simulink model "LinearMPC_pH"  (R2018a)
settings: Solver=ode45  StartTime=0.0  StopTime=10000  RelTol=1e-3  EnableMultiTasking=on
undefined symbols (not defined in the file or in its folder): sigbuilder_block
libraries: mpclib x1, simulink x1
settings Model: Creator=Debbie Ojigho  LastModifiedBy=Owolabi Israel
settings DataIOCC: LimitDataPoints=on  SaveFormat=Array
settings OptimizationCC: LifeSpan=inf
settings DebuggingCC: SFUnexpectedBacktrackingDiag=warning  SFNoUnconditionalDefaultTransitionDiag=warning  SFExecutionAtInitializationDiag=none
settings HardwareCC: ProdBitPerPointer=32  ProdBitPerSizeT=32  ProdBitPerPtrDiffT=32  ProdLargestAtomicFloat=None  ProdIntDivRoundTo=Undefined  ProdEndianess=Unspecified  ProdWordSize=32  ProdHWDeviceType=32-bit Generic
settings ModelReferenceCC: PropagateSignalLabelsOutOfModel=off
settings CodeAppCC: StateflowObjectComments=on
settings GRTTargetCC: TargetLangStandard=C89/C90 (ANSI)  GeneratePreprocessorConditionals=Disable all
settings ConfigComp: CovMetricSettings=dw  CovHtmlReporting=on  CovSaveCumulativeToWorkspaceVar=on  CovSaveSingleToWorkspaceVar=on  CovExternalEMLEnable=off

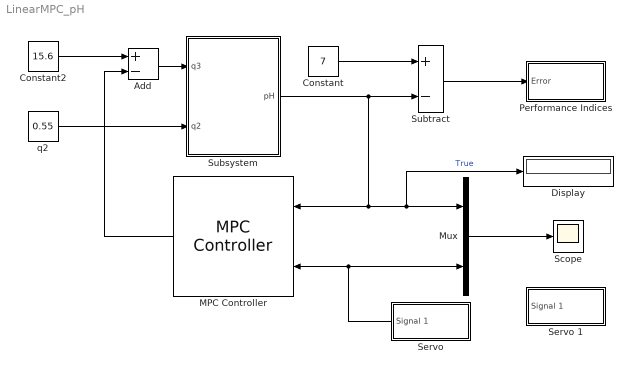
== system LinearMPC_pH ==
  Add : Sum  Inputs=+-
  Constant : Constant  Value=7
  Constant2 : Constant  Value=15.6
  Display : Display
  MPC Controller : mpclib/MPC Controller  SCDEnableBlockLinearizationSpecification=on  mpcobj=mpcobj_pH  x0=[]  is_multiple=0  enable_value=0  return_u0=off  updateMPCinCallerWorkspace=on  md_inport=off  mv_inport=off  uref_inport=off  cost_outport=off  return_sequence=off  return_qpstatus=off  return_xseq=off  return_state=off  return_ovseq=off  state_inport=off  umin_inport=off  umax_inport=off  ymin_inport=off  ymax_inport=off  cc_inport=off  ywt_inport=off  uwt_inport=off  duwt_inport=off  rhoeps_inport=off  pm_inport=off  MaximumP=10  HorizonChoice=FixedHorizon  n_ts=1  n_p=3  n_mv=1  n_md=0  n_ud=0  n_mo=1  n_uo=0  BlockDataType=double  SampleTimeInherited=off  switch_inport=off
      settings: SourceProductName=MATLAB Runtime - Model Predictive Control Toolbox Addin  SourceProductBaseCode=Missing
  Mux : Mux  Inputs=2
  Performance Indices : Subsystem
  Scope : Scope
  "Servo " : Subsystem  Tag=STV Subsys  LoadFcn=sigbuilder_block('load');  StartFcn=sigbuilder_block('start');  StopFcn=sigbuilder_block('stop');  ClipboardFcn=sigbuilder_block('clipboard');  mask(Sigbuilder block){tuvar=[0:10]}
      mask help: Sigbuilder GUI
      mask init:
      | if ~strcmp(get_param(bdroot(gcbh),'SimulationStatus'),'stopped') tuvar = sigbuilder_block('maskInit'); end
      settings: CopyFcn=sigbuilder_block('copy');  DeleteFcn=sigbuilder_block('delete');  ModelCloseFcn=sigbuilder_block('modelClose');  PreSaveFcn=sigbuilder_block('preSave');  PauseFcn=sigbuilder_block('pause')  ContinueFcn=sigbuilder_block('continue')  NameChangeFcn=sigbuilder_block('namechange');  OpenFcn=sigbuilder_block('open',[203.25 112.5 550.5 399.75 ]);  CloseFcn=sigbuilder_block('close');
      mask Display: plot(0, 0, 100, 100,[2, 2, 32, 32, 2], [68, 8, 8, 68, 68],[32, 2], [38, 38], [32, 19, 2],[53, 60, 44], [32, 17, 17, 2],[16, 16, 31, 31]);txt = getActiveGroup(gcbh);text(2, 100, txt,'verticalAlignment', 'top');
  Servo 1 : Subsystem  Tag=STV Subsys  LoadFcn=sigbuilder_block('load');  StartFcn=sigbuilder_block('start');  StopFcn=sigbuilder_block('stop');  ClipboardFcn=sigbuilder_block('clipboard');  mask(Sigbuilder block){tuvar=[0:10]}
      mask help: Sigbuilder GUI
      mask init:
      | if ~strcmp(get_param(bdroot(gcbh),'SimulationStatus'),'stopped') tuvar = sigbuilder_block('maskInit'); end
      settings: CopyFcn=sigbuilder_block('copy');  DeleteFcn=sigbuilder_block('delete');  ModelCloseFcn=sigbuilder_block('modelClose');  PreSaveFcn=sigbuilder_block('preSave');  PauseFcn=sigbuilder_block('pause')  ContinueFcn=sigbuilder_block('continue')  NameChangeFcn=sigbuilder_block('namechange');  OpenFcn=sigbuilder_block('open',[203.25 112.5 550.5 399.75 ]);  CloseFcn=sigbuilder_block('close');
      mask Display: plot(0, 0, 100, 100,[2, 2, 32, 32, 2], [68, 8, 8, 68, 68],[32, 2], [38, 38], [32, 19, 2],[53, 60, 44], [32, 17, 17, 2],[16, 16, 31, 31]);txt = getActiveGroup(gcbh);text(2, 100, txt,'verticalAlignment', 'top');
  Subsystem : Subsystem
  Subtract : Sum  Inputs=+-
  q2 : Constant  Value=0.55
  wires:
  Subtract/1 -> Performance Indices/1("Error ")
  Mux/1 -> Scope/1
  Subsystem/1(pH) -> Subtract/2, MPC Controller/1, Display/1, Mux/1  "True"
  Constant/1 -> Subtract/1
  "Servo "/1(Signal 1) -> MPC Controller/2, Mux/2
  q2/1 -> Subsystem/2(q2)
  Add/1 -> Subsystem/1(q3)
  Constant2/1 -> Add/1
  MPC Controller/1 -> Add/2

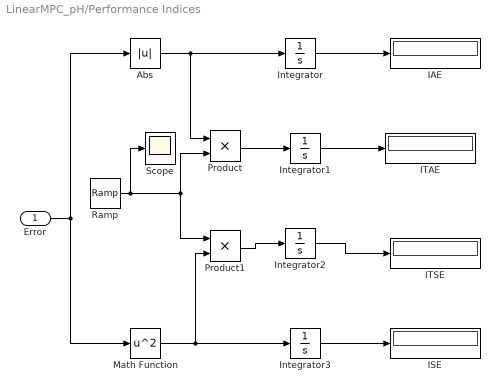
== system LinearMPC_pH/Performance Indices ==
  "Error " : Inport
  Abs : Abs
  IAE : Display
  ISE : Display
  ITAE : Display
  ITSE : Display
  Integrator{,1..3} (4 alike) : Integrator
  Math Function : Math  Operator=square  SaturateOnIntegerOverflow=on
  Product : Product  RndMeth=Zero
  Product1 : Product  RndMeth=Zero
  Ramp : simulink/Sources/Ramp  slope=1  start=0  InitialOutput=0
  Scope : Scope
  wires:
  "Error "/1 -> Math Function/1, Abs/1
  Abs/1 -> Integrator/1, Product/1
  Integrator/1 -> IAE/1
  Ramp/1 -> Product/2, Product1/1, Scope/1
  Math Function/1 -> Integrator3/1, Product1/2
  Product1/1 -> Integrator2/1
  Product/1 -> Integrator1/1
  Integrator3/1 -> ISE/1
  Integrator2/1 -> ITSE/1
  Integrator1/1 -> ITAE/1

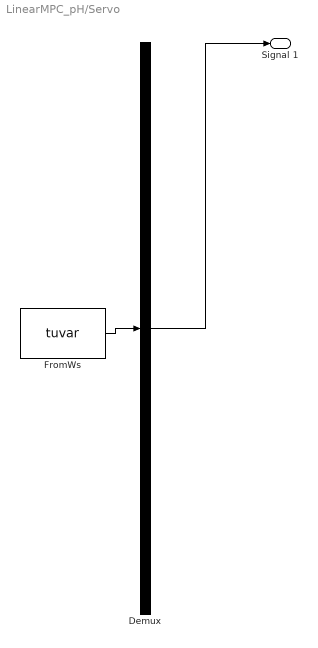
== system LinearMPC_pH/Servo  ==
  Demux : Demux  Tag=STV Demux  Outputs=1
  FromWs : FromWorkspace  Tag=STV FromWs  VariableName=tuvar  SampleTime=0
      SigBuilderData=|
      | common.afterFinalStr = 'Extrapolate'
      | common.sampleTime = 0
      | dataSet.timeRange = [0 10000]
      | dataSet.name = 'pH Signal'
      | sbobj.Groups.Name = 'pH Signal'
      | sbobj.Groups.Signals.Name = 'Signal 1'
      | sbobj.Groups.Signals.XData = [0 2000 2000 4000 4000 6000 6000 8000 8000 10000]
      | sbobj.Groups.Signals.YData = [4 4 5 5 6 6 7 7 6 6]
      | sbobj.Groups.TimeRange = [0 10000]
  Signal 1 : Outport  Tag=STV Outport
  wires:
  Demux/1 -> Signal 1/1
  FromWs/1 -> Demux/1

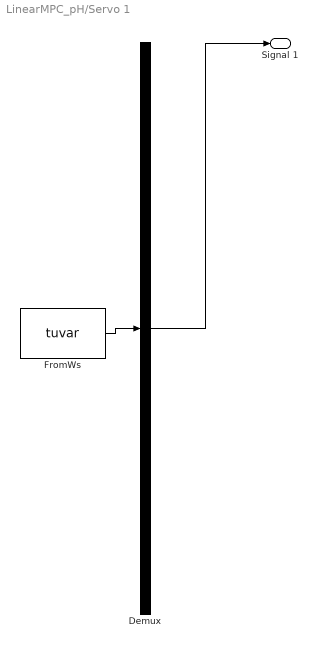
== system LinearMPC_pH/Servo 1 ==
  Demux : Demux  Tag=STV Demux  Outputs=1
  FromWs : FromWorkspace  Tag=STV FromWs  VariableName=tuvar  SampleTime=0
      SigBuilderData=|
      | common.afterFinalStr = 'Extrapolate'
      | common.sampleTime = 0
      | dataSet.timeRange = [0 6000]
      | dataSet.name = 'pH Signal'
      | sbobj.Groups.Name = 'pH Signal'
      | sbobj.Groups.Signals.Name = 'Signal 1'
      | sbobj.Groups.Signals.XData = [0 1000 1000 2000 2000 3000 3000 4000 4000 5000 5000 6000]
      | sbobj.Groups.Signals.YData = [6.5 6.5 7 7 7.5 7.5 7 7 6.5 6.5 7 7]
      | sbobj.Groups.TimeRange = [0 6000]
  Signal 1 : Outport  Tag=STV Outport
  wires:
  Demux/1 -> Signal 1/1
  FromWs/1 -> Demux/1

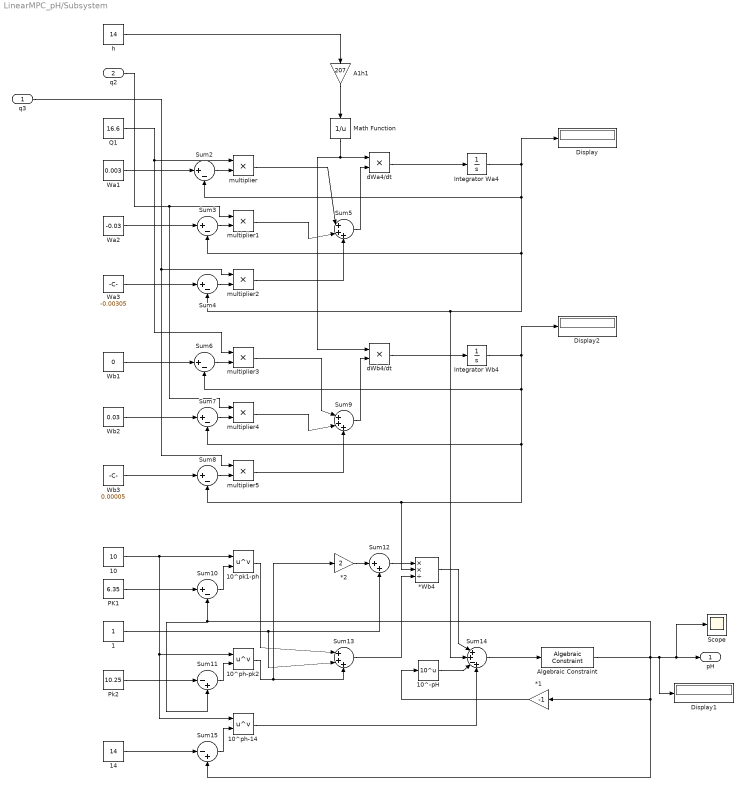
== system LinearMPC_pH/Subsystem ==
  q3 : Inport
  q2 : Inport  Port=2
  *1 : Gain  Gain=-1
  *2 : Gain  Gain=2
  *Wb4 : Product  Inputs=**/
  1 : Constant
  10 : Constant  Value=10
  10^-pH : Math  Operator=10^u  SaturateOnIntegerOverflow=on
  10^ph-14 : Math  Operator=pow  SaturateOnIntegerOverflow=on
  10^ph-pk2 : Math  Operator=pow  SaturateOnIntegerOverflow=on
  10^pk1-ph : Math  Operator=pow  SaturateOnIntegerOverflow=on
  14 : Constant  Value=14
  A1h1 : Gain  Gain=207
  Algebraic Constraint : AlgebraicConstraint  InitialGuess=7
  Display : Display
  Display1 : Display
  Display2 : Display
  Integrator Wa4 : Integrator  InitialCondition=-0.000432
  Integrator Wb4 : Integrator  InitialCondition=0.000528
  Math Function : Math  Operator=reciprocal  SaturateOnIntegerOverflow=on
  PK1 : Constant  Value=6.35
  Pk2 : Constant  Value=10.25
  Q1 : Constant  Value=16.6
  Scope : Scope
  Sum{2..4,6..8,10} (7 alike) : Sum  Inputs=|+-
  Sum11 : Sum  Inputs=|-+
  Sum12 : Sum  Inputs=|++
  Sum13 : Sum  Inputs=|+++
  Sum14 : Sum  Inputs=|++-+
  Sum15 : Sum  Inputs=|-+
  Sum5 : Sum  Inputs=|+++
  Sum9 : Sum  Inputs=|+++
  Wa1 : Constant  Value=0.003
  Wa2 : Constant  Value=-0.03
  Wa3 : Constant  Value=-0.00305
  Wb1 : Constant  Value=0
  Wb2 : Constant  Value=0.03
  Wb3 : Constant  Value=0.00005
  dWa4/dt : Product
  dWb4/dt : Product
  h : Constant  Value=14
  multiplier{,1..5} (6 alike) : Product
  pH : Outport
  wires:
  q2/1 -> multiplier4/1, multiplier1/1
  Sum15/1 -> 10^ph-14/2
  14/1 -> Sum15/1
  Sum3/1 -> multiplier1/2
  Sum5/1 -> dWa4/dt/2
  Wb1/1 -> Sum6/1
  Wb3/1 -> Sum8/1
  Wa1/1 -> Sum2/1
  Sum8/1 -> multiplier5/2
  multiplier4/1 -> Sum9/2
  10^ph-14/1 -> Sum14/4
  1/1 -> Sum13/2, Sum12/2
  Wb2/1 -> Sum7/1
  Math Function/1 -> dWa4/dt/1, dWb4/dt/1
  multiplier3/1 -> Sum9/1
  *1/1 -> 10^-pH/1
  10/1 -> 10^ph-pk2/1, 10^ph-14/1, 10^pk1-ph/1
  Sum10/1 -> 10^pk1-ph/2
  Sum13/1 -> *Wb4/3
  Pk2/1 -> Sum11/1
  Sum11/1 -> 10^ph-pk2/2
  Sum12/1 -> *Wb4/1
  Sum14/1 -> Algebraic Constraint/1
  Wa3/1 -> Sum4/1
  multiplier2/1 -> Sum5/3
  10^-pH/1 -> Sum14/3
  A1h1/1 -> Math Function/1
  Q1/1 -> multiplier3/1, multiplier/1
  PK1/1 -> Sum10/1
  multiplier5/1 -> Sum9/3
  10^ph-pk2/1 -> *2/1, Sum13/3
  Integrator Wb4/1 -> Display2/1, Sum6/2, Sum7/2, *Wb4/2, Sum8/2
  Algebraic Constraint/1 -> Sum11/2, Sum10/2, Display1/1, Scope/1, pH/1, *1/1, Sum15/2
  multiplier/1 -> Sum5/1
  dWa4/dt/1 -> Integrator Wa4/1
  *Wb4/1 -> Sum14/1
  h/1 -> A1h1/1
  multiplier1/1 -> Sum5/2
  Sum9/1 -> dWb4/dt/2
  *2/1 -> Sum12/1
  Integrator Wa4/1 -> Display/1, Sum2/2, Sum3/2, Sum14/2, Sum4/2
  Sum2/1 -> multiplier/2
  Sum7/1 -> multiplier4/2
  Sum6/1 -> multiplier3/2
  10^pk1-ph/1 -> Sum13/1
  Sum4/1 -> multiplier2/2
  dWb4/dt/1 -> Integrator Wb4/1
  Wa2/1 -> Sum3/1
  q3/1 -> multiplier5/1, multiplier2/1
